simulink library "slctrlblks"  (Simulink 7.6)
settings: Solver=ode45  SolverMode=SingleTasking  StartTime=0.0  StopTime=10.0  RelTol=1e-3
undefined symbols (not defined in the file or in its folder): slctrlblkdlgs
libraries: slctrlextras x12, slctrlblks x6
settings Model: Creator=jglass  LastModifiedBy=astother

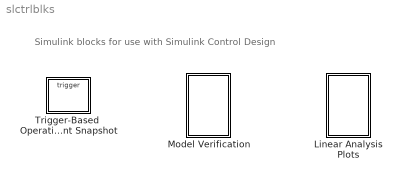
== system slctrlblks ==
  note: Simulink blocks for use with Simulink Control Design
  Linear Analysis Plots : Subsystem
  Model Verification : Subsystem
  Trigger-Based  Operating Point Snapshot : Subsystem  TreatAsAtomicUnit=on  mask(Triggered Operating Condition/Linearization Snapshot){TriggerType=rising}
      mask prompts: TriggerType "Trigger type:"
      mask help: Generate operating points and/or linearizations at triggered events
      mask init:
      | set_param([ gcb '/Trigger'],'TriggerType',TriggerType);
      mask Help: eval('scdguihelp(''trigger_based_operating_point_snapshot_block'',''HelpBrowser'')')
      mask StyleString: popup(rising|falling|either|function-call)

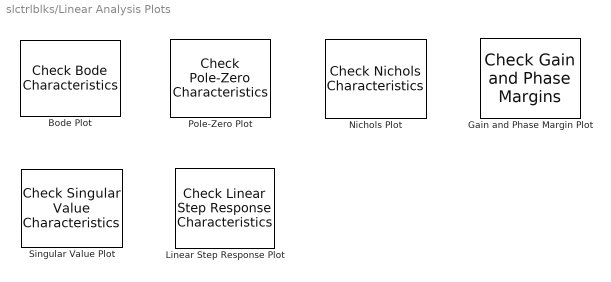
== system slctrlblks/Linear Analysis Plots ==
  Bode Plot : slctrlblks/Model Verification/Check Bode  Characteristics  DialogController=checkpack.createCheckDlg  DialogControllerArgs=DataTag0  SystemSampleTime=-1  LinearizationIOs={}  LinearizeAt=SnapshotTimes  SnapshotTimes=[0]  TriggerType=rising  SampleTime=auto  RateConversionMethod=zoh  PreWarpFreq=10  UseExactDelayModel=off  UseFullBlockNameLabels=off  UseBusSignalLabels=off  enabled=on  stopWhenAssertionFail=off  export=off  ViewDlgPos=[]  OpenViewOnLoad=off  LaunchViewOnOpen=off  EnableUpperBound=off  UpperBoundFrequencies=[]  UpperBoundMagnitudes=[]  EnableLowerBound=off  LowerBoundFrequencies=[]  LowerBoundMagnitudes=[]
  Gain and Phase Margin Plot : slctrlblks/Model Verification/Check Gain and Phase Margins  DialogController=checkpack.createCheckDlg  DialogControllerArgs=DataTag1  SystemSampleTime=-1  LinearizationIOs={}  LinearizeAt=SnapshotTimes  SnapshotTimes=[0]  TriggerType=rising  SampleTime=auto  RateConversionMethod=zoh  PreWarpFreq=10  UseExactDelayModel=off  UseFullBlockNameLabels=off  UseBusSignalLabels=off  enabled=on  stopWhenAssertionFail=off  export=off  ViewDlgPos=[]  LaunchViewOnOpen=off  OpenViewOnLoad=off  EnableMargins=off  GainMargin=[]  PhaseMargin=[]  PlotType=bode  FeedbackSign=-1
      settings: SaveToWorkspace=off  SaveName=sys
  Linear Step Response Plot : slctrlblks/Model Verification/Check Linear Step Response Characteristics  DialogController=checkpack.createCheckDlg  DialogControllerArgs=DataTag2  SystemSampleTime=-1  LinearizationIOs={}  LinearizeAt=SnapshotTimes  SnapshotTimes=[0]  TriggerType=rising  SampleTime=auto  RateConversionMethod=zoh  PreWarpFreq=10  UseExactDelayModel=off  UseFullBlockNameLabels=off  UseBusSignalLabels=off  enabled=on  stopWhenAssertionFail=off  export=off  ViewDlgPos=[]  OpenViewOnLoad=off  LaunchViewOnOpen=off  EnableStepResponseBound=off  FinalValue=[]  RiseTime=[]  PercentRise=[]  SettlingTime=[]  PercentSettling=[]  PercentOvershoot=[]  PercentUndershoot=[]
      settings: SaveToWorkspace=off  SaveName=sys
  Nichols Plot : slctrlblks/Model Verification/Check Nichols Characteristics  DialogController=checkpack.createCheckDlg  DialogControllerArgs=DataTag3  SystemSampleTime=-1  LinearizationIOs={}  LinearizeAt=SnapshotTimes  SnapshotTimes=[0]  TriggerType=rising  SampleTime=auto  RateConversionMethod=zoh  PreWarpFreq=10  UseExactDelayModel=off  UseFullBlockNameLabels=off  UseBusSignalLabels=off  enabled=on  stopWhenAssertionFail=off  export=off  ViewDlgPos=[]  LaunchViewOnOpen=off  OpenViewOnLoad=off  EnableMargins=off  GainMargin=[]  PhaseMargin=[]  EnableGainPhaseBound=off  GainPhaseBoundType={'upper'}  OLPhases=[]  OLGains=[]  EnableCLPeakGain=off  CLPeakGain=[]  FeedbackSign=-1
      settings: SaveToWorkspace=off  SaveName=sys
  Pole-Zero Plot : slctrlblks/Model Verification/Check Pole-Zero Characteristics  DialogController=checkpack.createCheckDlg  DialogControllerArgs=DataTag4  SystemSampleTime=-1  LinearizationIOs={}  LinearizeAt=SnapshotTimes  SnapshotTimes=[0]  TriggerType=rising  SampleTime=auto  RateConversionMethod=zoh  PreWarpFreq=10  UseExactDelayModel=off  UseFullBlockNameLabels=off  UseBusSignalLabels=off  enabled=on  stopWhenAssertionFail=off  export=off  ViewDlgPos=[]  LaunchViewOnOpen=off  OpenViewOnLoad=off  EnableSettlingTime=off  SettlingTime=[]  EnablePercentOvershoot=off  PercentOvershoot=[]  EnableDampingRatio=off  DampingRatio=[]  EnableNaturalFrequency=off  NaturalFrequencyBound=>=  NaturalFrequency=[]
      settings: SaveToWorkspace=off  SaveName=sys
  Singular Value Plot : slctrlblks/Model Verification/Check Singular Value Characteristics  DialogController=checkpack.createCheckDlg  DialogControllerArgs=DataTag5  SystemSampleTime=-1  LinearizationIOs={}  LinearizeAt=SnapshotTimes  SnapshotTimes=[0]  TriggerType=rising  SampleTime=auto  RateConversionMethod=zoh  PreWarpFreq=10  UseExactDelayModel=off  UseFullBlockNameLabels=off  UseBusSignalLabels=off  enabled=on  stopWhenAssertionFail=off  export=off  LaunchViewOnOpen=off  ViewDlgPos=[]  OpenViewOnLoad=off  EnableUpperBound=off  UpperBoundFrequencies=[]  UpperBoundMagnitudes=[]  EnableLowerBound=off  LowerBoundFrequencies=[]  LowerBoundMagnitudes=[]
      settings: SaveToWorkspace=off  SaveName=sys

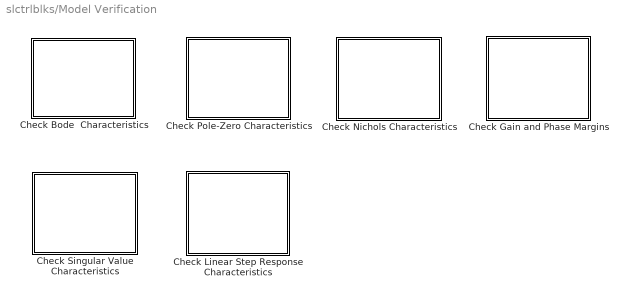
== system slctrlblks/Model Verification ==
  Check Bode  Characteristics : Subsystem  InstantiateOnLoad=on  DialogController=checkpack.createCheckDlg  DialogControllerArgs=DataTag6  LoadFcn=slctrlblkdlgs.absCheckFrequencyDlg.loadBlkFcn(gcb)  mask(Checks_Bode){SaveToWorkspace=off, SaveName=sys, LinearizationIOs={}, LinearizeAt=SnapshotTimes, SnapshotTimes=[0], TriggerType=rising, ZeroCross=on, SampleTime=auto, RateConversionMethod=zoh, PreWarpFreq=10, UseExactDelayModel=off, UseFullBlockNameLabels=off, UseBusSignalLabels=off, enabled=on, callback=, stopWhenAssertionFail=off, export=off, ViewDlgPos=[], OpenViewOnLoad=off, LaunchViewOnOpen=off, FrequencyUnits=, MagnitudeUnits=, PhaseUnits=, EnableUpperBound=on, UpperBoundFrequencies=[10 100], UpperBoundMagnitudes=[-20 -20], EnableLowerBound=on, LowerBoundFrequencies=[0.1 1], LowerBoundMagnitudes=[20 20]}
      mask prompts: SaveToWorkspace "Save data to workspace"; SaveName "Variable name:"; LinearizationIOs "Linearization IOs"; LinearizeAt "Linearize:"; SnapshotTimes "Snapshot times:"; TriggerType "Trigger type:"; ZeroCross "Enable zero-crossing detection"; SampleTime "Sample time:"; RateConversionMethod "Sample time conversion method"; PreWarpFreq "Prewarp frequency"; UseExactDelayModel "Use exact delays"; UseFullBlockNameLabels "Use full block name to label model I/O"; UseBusSignalLabels "Use bus signal nems to label model IO"; enabled "Enable assertion"; callback "Simulation callback when assertion fails (optional):"; stopWhenAssertionFail "Stop simulation when assertion fails"; export "Output assertion signal"; OpenViewOnLoad "Open view when loading"; LaunchViewOnOpen "Launch view on open"; EnableUpperBound "Upper magnitude bound"; UpperBoundFrequencies "Frequencies (Hz):"; UpperBoundMagnitudes "Magnitudes (db):"; EnableLowerBound "Lower magnitude bound"; LowerBoundFrequencies "Frequencies (Hz):"; LowerBoundMagnitudes "Magnitudes (db):"
      mask init:
      | slctrlblkdlgs.CheckBodeDlg.configBlk(gcbh)
      settings: CopyFcn=slctrlblkdlgs.absCheckFrequencyDlg.copyBlkFcn(gcb)  OpenFcn=checkpack.absCheckDlg.openBlkFcn(gcbh)
      mask Help: eval('scdguihelp(''bode_plot_block'',''HelpBrowser'')')
      mask StyleString: checkbox,edit,edit,popup(SnapshotTimes|ExternalTrigger),edit,popup(rising|falling),checkbox,edit,popup(zoh|tustin|prewarp|upsampling_zoh|upsampling_tustin|upsampling_prewarp),edit,checkbox,checkbox,checkbox,checkbox,edit,checkbox,checkbox,edit,checkbox,checkbox,edit,edit,edit,checkbox,edit,edit,checkbox,edit,edit
      mask TabNameString: Logging,Logging,Linearizations,Linearizations,Linearizations,Linearizations,Linearizations,Linearizations,Linearizations,Linearizations,Linearizations,Linearizations,Linearizations,Assertion,Assertion,Assertion,Assertion,Misc.,Misc.,Misc,Misc,Misc,Misc,Bounds,Bounds,Bounds,Bounds,Bounds,Bounds
      mask Display: image(imread('C:\Sandbox\Acontrol_08042010\matlab\toolbox\slcontrol\slctrlutil\resources\CheckBodeIcon.bmp','bmp'),'center');
  Check Gain and Phase Margins : Subsystem  InstantiateOnLoad=on  DialogController=checkpack.createCheckDlg  DialogControllerArgs=DataTag7  LoadFcn=slctrlblkdlgs.absCheckFrequencyDlg.loadBlkFcn(gcb)  mask(Checks_Margins){SaveToWorkspace=off, SaveName=sys, LinearizationIOs={}, LinearizeAt=SnapshotTimes, SnapshotTimes=[0], TriggerType=rising, ZeroCross=on, SampleTime=auto, RateConversionMethod=zoh, PreWarpFreq=10, UseExactDelayModel=off, UseFullBlockNameLabels=off, UseBusSignalLabels=off, enabled=on, callback=, stopWhenAssertionFail=off, export=off, ViewDlgPos=[], LaunchViewOnOpen=off, OpenViewOnLoad=off, FrequencyUnits=, MagnitudeUnits=, PhaseUnits=, EnableMargins=on, GainMargin=20, PhaseMargin=30, PlotType=bode, FeedbackSign=-1}
      mask prompts: SaveToWorkspace "Save data to workspace"; SaveName "Variable name:"; LinearizationIOs "Linearization IOs"; LinearizeAt "Linearize:"; SnapshotTimes "Snapshot times:"; TriggerType "Trigger type:"; ZeroCross "Enable zero-crossing detection"; SampleTime "Sample time:"; RateConversionMethod "Sample time rate conversion method"; PreWarpFreq "Prewarp frequency"; UseExactDelayModel "Use exact delays"; UseFullBlockNameLabels "Use full block name to label model I/O"; UseBusSignalLabels "Use bus signal names to label model I/O"; enabled "Enable assertion"; callback "Simulation callback when assertion fails"; stopWhenAssertionFail "Stop simulation when assertion fails"; export "Output assertion signal"; LaunchViewOnOpen "Launch view on open"; OpenViewOnLoad "Open view when loading"; EnableMargins "Enforce Gain & Phase margins"; GainMargin "Gain margin (db) >"; PhaseMargin "Phase margin (deg) >"; PlotType "Plot type"; FeedbackSign "Feedback sign"
      mask init:
      | slctrlblkdlgs.CheckMarginsDlg.configBlk(gcbh)
      settings: CopyFcn=slctrlblkdlgs.absCheckFrequencyDlg.copyBlkFcn(gcb)  OpenFcn=checkpack.absCheckDlg.openBlkFcn(gcbh)
      mask Help: eval('scdguihelp(''gain_phase_margin_plot_block'',''HelpBrowser'')')
      mask StyleString: checkbox,edit,edit,popup(SnapshotTimes|ExternalTrigger),edit,popup(rising|falling),checkbox,edit,popup(zoh|tustin|prewarp|upsampling_zoh|upsampling_tustin|upsampling_prewarp),edit,checkbox,checkbox,checkbox,checkbox,edit,checkbox,checkbox,edit,checkbox,checkbox,edit,edit,edit,checkbox,edit,edit,popup(bode|nichols|nyquist|table),popup(-1|+1)
      mask TabNameString: Logging,Logging,Linearizations,Linearizations,Linearizations,Linearizations,Linearizations,Linearizations,Linearizations,Linearizations,Linearizations,Linearizations,Linearizations,Assertion,Assertion,Assertion,Assertion,Misc,Misc,Misc,Misc,Misc,Misc,Bounds,Bounds,Bounds,Bounds,Bounds
      mask Display: image(imread('C:\Sandbox\Acontrol_08042010\matlab\toolbox\slcontrol\slctrlutil\resources\CheckMarginsIcon.bmp','bmp'),'center');
  Check Linear Step Response Characteristics : Subsystem  InstantiateOnLoad=on  DialogController=checkpack.createCheckDlg  DialogControllerArgs=DataTag8  LoadFcn=slctrlblkdlgs.absCheckFrequencyDlg.loadBlkFcn(gcb)  mask(Checks_LinearStepResponse){SaveToWorkspace=off, SaveName=sys, LinearizationIOs={}, LinearizeAt=SnapshotTimes, SnapshotTimes=[0], TriggerType=rising, ZeroCross=on, SampleTime=auto, RateConversionMethod=zoh, PreWarpFreq=10, UseExactDelayModel=off, UseFullBlockNameLabels=off, UseBusSignalLabels=off, enabled=on, callback=, stopWhenAssertionFail=off, export=off, ViewDlgPos=[], OpenViewOnLoad=off, LaunchViewOnOpen=off, FrequencyUnits=, MagnitudeUnits=, PhaseUnits=, EnableStepResponseBound=on, FinalValue=1, RiseTime=5, PercentRise=80, SettlingTime=7, PercentSettling=1, PercentOvershoot=10, PercentUndershoot=1}
      mask prompts: SaveToWorkspace "Save data to workspace"; SaveName "Variable name:"; LinearizationIOs "Linearization IOs"; LinearizeAt "Linearize:"; SnapshotTimes "Snapshot times:"; TriggerType "Trigger type:"; ZeroCross "Enable zero-crossing detection"; SampleTime "Sample time:"; RateConversionMethod "Sample time conversion method"; PreWarpFreq "Prewarp frequency"; UseExactDelayModel "Use exact delays"; UseFullBlockNameLabels "Use full block name to label Model I/Os"; UseBusSignalLabels "Use bus signal names to label model I/Os"; enabled "Enable assertion"; callback "Simulation callback when assertion fails"; stopWhenAssertionFail "Stop simulation when assertion fails"; export "Output assertion signal"; OpenViewOnLoad "Open view when loading"; LaunchViewOnOpen "Launch view on open"; EnableStepResponseBound "Enforce Step Response bound"; FinalValue "Final step value:"; RiseTime "Rise time:"; PercentRise "Percentage rise:"; SettlingTime "Settling time:"; PercentSettling "Percentage settling:"; PercentOvershoot "Percentage overshoot:"; PercentUndershoot "Percentage undershoot:"
      mask init:
      | slctrlblkdlgs.CheckLinStepDlg.configBlk(gcbh)
      settings: CopyFcn=slctrlblkdlgs.absCheckFrequencyDlg.copyBlkFcn(gcb)  OpenFcn=checkpack.absCheckDlg.openBlkFcn(gcbh)
      mask Help: eval('scdguihelp(''step_response_plot_block'',''HelpBrowser'')')
      mask StyleString: checkbox,edit,edit,popup(SnapshotTimes|ExternalTrigger),edit,popup(rising|falling),checkbox,edit,popup(zoh|tustin|prewarp|upsampling_zoh|upsampling_tustin|upsampling_prewarp),edit,checkbox,checkbox,checkbox,checkbox,edit,checkbox,checkbox,edit,checkbox,checkbox,edit,edit,edit,checkbox,edit,edit,edit,edit,edit,edit,edit
      mask TabNameString: Logging,Logging,Linearizations,Linearizations,Linearizations,Linearizations,Linearizations,Linearizations,Linearizations,Linearizations,Linearizations,Linearizations,Linearizations,Assertion,Assertion,Assertion,Assertion,Misc,Misc,Misc,Misc,Misc,Misc,Bounds,Bounds,Bounds,Bounds,Bounds,Bounds,Bounds,Bounds
      mask Display: image(imread('C:\Sandbox\Acontrol_08042010\matlab\toolbox\slcontrol\slctrlutil\resources\CheckLinStepIcon.bmp','bmp'),'center');
  Check Nichols Characteristics : Subsystem  InstantiateOnLoad=on  DialogController=checkpack.createCheckDlg  DialogControllerArgs=DataTag9  LoadFcn=slctrlblkdlgs.absCheckFrequencyDlg.loadBlkFcn(gcb)  mask(Checks_Nichols){SaveToWorkspace=off, SaveName=sys, LinearizationIOs={}, LinearizeAt=SnapshotTimes, SnapshotTimes=[0], TriggerType=rising, ZeroCross=on, SampleTime=auto, RateConversionMethod=zoh, PreWarpFreq=10, UseExactDelayModel=off, UseFullBlockNameLabels=off, UseBusSignalLabels=off, enabled=on, callback=, stopWhenAssertionFail=off, export=off, ViewDlgPos=[], LaunchViewOnOpen=off, OpenViewOnLoad=off, FrequencyUnits=, MagnitudeUnits=, PhaseUnits=, EnableMargins=on, GainMargin=20, PhaseMargin=30, EnableGainPhaseBound=off, GainPhaseBoundType={'upper'}, OLPhases=[], OLGains=[], EnableCLPeakGain=off, CLPeakGain=[], FeedbackSign=-1}
      mask prompts: SaveToWorkspace "Save data to workspace"; SaveName "Variable name:"; LinearizationIOs "Linearization IOs"; LinearizeAt "Linearize:"; SnapshotTimes "Snapshot times:"; TriggerType "Trigger type:"; ZeroCross "Enable zero-crossing detection"; SampleTime "Sample time:"; RateConversionMethod "Sample time conversion method"; PreWarpFreq "Prewarp frequency"; UseExactDelayModel "Use exact delays"; UseFullBlockNameLabels "Use full block name to label model I/O"; UseBusSignalLabels "Use bus signal names to label model I/O"; enabled "Enable assertion"; callback "Simulation callback when assertion fails"; stopWhenAssertionFail "Stop simulation when assertion fails"; export "Output assertion signal"; LaunchViewOnOpen "Launch view on open"; OpenViewOnLoad "Open view when loading"; EnableMargins "Enforce Gain & Phase margins"; GainMargin "Gain margin (db) >"; PhaseMargin "Phase margin (deg) >"; EnableGainPhaseBound "Gain-Phase bound"; GainPhaseBoundType "Type:"; OLPhases "Open-loop phases (deg)"; OLGains "Open-loop gains (db)"; EnableCLPeakGain "Closed-loop peak gain bound"; CLPeakGain "Closed-loop peak gain (db) <"; FeedbackSign "Feedback sign"
      mask init:
      | slctrlblkdlgs.CheckNicholsDlg.configBlk(gcbh)
      settings: CopyFcn=slctrlblkdlgs.absCheckFrequencyDlg.copyBlkFcn(gcb)  OpenFcn=checkpack.absCheckDlg.openBlkFcn(gcbh)
      mask Help: eval('scdguihelp(''nichols_plot_block'',''HelpBrowser'')')
      mask StyleString: checkbox,edit,edit,popup(SnapshotTimes|ExternalTrigger),edit,popup(rising|falling),checkbox,edit,popup(zoh|tustin|prewarp|upsampling_zoh|upsampling_tustin|upsampling_prewarp),edit,checkbox,checkbox,checkbox,checkbox,edit,checkbox,checkbox,edit,checkbox,checkbox,edit,edit,edit,checkbox,edit,edit,checkbox,edit,edit,edit,checkbox,edit,popup(-1|+1)
      mask TabNameString: Logging,Logging,Linearizations,Linearizations,Linearizations,Linearizations,Linearizations,Linearizations,Linearizations,Linearizations,Linearizations,Linearizations,Linearizations,Assertion,Assertion,Assertion,Assertion,Misc,Misc,Misc,Misc,Misc,Misc,Bounds,Bounds,Bounds,Bounds,Bounds,Bounds,Bounds,Bounds,Bounds,Bounds
      mask Display: image(imread('C:\Sandbox\Acontrol_08042010\matlab\toolbox\slcontrol\slctrlutil\resources\CheckNicholsIcon.bmp','bmp'),'center');
  Check Pole-Zero Characteristics : Subsystem  InstantiateOnLoad=on  DialogController=checkpack.createCheckDlg  DialogControllerArgs=DataTag10  LoadFcn=slctrlblkdlgs.absCheckFrequencyDlg.loadBlkFcn(gcb)  mask(Checks_PZMap){SaveToWorkspace=off, SaveName=sys, LinearizationIOs={}, LinearizeAt=SnapshotTimes, SnapshotTimes=[0], TriggerType=rising, ZeroCross=on, SampleTime=auto, RateConversionMethod=zoh, PreWarpFreq=10, UseExactDelayModel=off, UseFullBlockNameLabels=off, UseBusSignalLabels=off, enabled=on, callback=, stopWhenAssertionFail=off, export=off, ViewDlgPos=[], LaunchViewOnOpen=off, OpenViewOnLoad=off, FrequencyUnits=, MagnitudeUnits=, PhaseUnits=, EnableSettlingTime=on, SettlingTime=1, EnablePercentOvershoot=on, PercentOvershoot=10, EnableDampingRatio=off, DampingRatio=[], EnableNaturalFrequency=off, NaturalFrequencyBound=>=, NaturalFrequency=[]}
      mask prompts: SaveToWorkspace "Save data to workspace"; SaveName "Variable name:"; LinearizationIOs "Linearization IOs"; LinearizeAt "Linearize:"; SnapshotTimes "Snapshot times:"; TriggerType "Trigger type:"; ZeroCross "Enable zero-crossing detection"; SampleTime "Sample time:"; RateConversionMethod "Sample time conversion method"; PreWarpFreq "Prewarp frequency"; UseExactDelayModel "Use exact delays"; UseFullBlockNameLabels "Use full block name to label model I/O"; UseBusSignalLabels "Use bus signal names to label model I/O"; enabled "Enable assertion"; callback "Simulation callback when assertion fails"; stopWhenAssertionFail "Stop simulation when assertion fails"; export "Output assertion signal"; LaunchViewOnOpen "Launch view on open"; OpenViewOnLoad "Open view when loading"; EnableSettlingTime "Settling time bound"; SettlingTime "Settling time (sec) <"; EnablePercentOvershoot "Overshoot bound"; PercentOvershoot "Percent overshoot <"; EnableDampingRatio "Damping ratio bound"; DampingRatio "Damping ratio <"; EnableNaturalFrequency "Natural frequency bound"; NaturalFrequencyBound "Natural frequency bound type"; NaturalFrequency "Natural frequency"
      mask init:
      | slctrlblkdlgs.CheckPZMapDlg.configBlk(gcbh)
      settings: CopyFcn=slctrlblkdlgs.absCheckFrequencyDlg.copyBlkFcn(gcb)  OpenFcn=checkpack.absCheckDlg.openBlkFcn(gcbh)
      mask Help: eval('scdguihelp(''pole_zero_plot_block'',''HelpBrowser'')')
      mask StyleString: checkbox,edit,edit,popup(SnapshotTimes|ExternalTrigger),edit,popup(rising|falling),checkbox,edit,popup(zoh|tustin|prewarp|upsampling_zoh|upsampling_tustin|upsampling_prewarp),edit,checkbox,checkbox,checkbox,checkbox,edit,checkbox,checkbox,edit,checkbox,checkbox,edit,edit,edit,checkbox,edit,checkbox,edit,checkbox,edit,checkbox,popup(>=|<=),edit
      mask TabNameString: Logging,Logging,Linearizations,Linearizations,Linearizations,Linearizations,Linearizations,Linearizations,Linearizations,Linearizations,Linearizations,Linearizations,Linearizations,Assertion,Assertion,Assertion,Assertion,Misc.,Misc.,Misc.,Misc.,Misc.,Misc.,Bounds,Bounds,Bounds,Bounds,Bounds,Bounds,Bounds,Bounds,Bounds
      mask Display: image(imread('C:\Sandbox\Acontrol_08042010\matlab\toolbox\slcontrol\slctrlutil\resources\CheckPZMapIcon.bmp','bmp'),'center');
  Check Singular Value Characteristics : Subsystem  InstantiateOnLoad=on  DialogController=checkpack.createCheckDlg  DialogControllerArgs=DataTag11  LoadFcn=slctrlblkdlgs.absCheckFrequencyDlg.loadBlkFcn(gcb)  mask(Checks_Sigma){SaveToWorkspace=off, SaveName=sys, LinearizationIOs={}, LinearizeAt=SnapshotTimes, SnapshotTimes=[0], TriggerType=rising, ZeroCross=on, SampleTime=auto, RateConversionMethod=zoh, PreWarpFreq=10, UseExactDelayModel=off, UseFullBlockNameLabels=off, UseBusSignalLabels=off, enabled=on, callback=, stopWhenAssertionFail=off, export=off, LaunchViewOnOpen=off, ViewDlgPos=[], OpenViewOnLoad=off, FrequencyUnits=, MagnitudeUnits=, PhaseUnits=, EnableUpperBound=on, UpperBoundFrequencies=[0.1 100], UpperBoundMagnitudes=[0 0], EnableLowerBound=off, LowerBoundFrequencies=[], LowerBoundMagnitudes=[]}
      mask prompts: SaveToWorkspace "Save data to workspace"; SaveName "Variable name:"; LinearizationIOs "Linearization IOs"; LinearizeAt "Linearize:"; SnapshotTimes "Snapshot times:"; TriggerType "Trigger type:"; ZeroCross "Enable zero-crossing detection"; SampleTime "Sample time:"; RateConversionMethod "Sample time conversion method"; PreWarpFreq "Prewarp frequency"; UseExactDelayModel "Use exact delays"; UseFullBlockNameLabels "Use full block name to label model I/Os"; UseBusSignalLabels "Use bus signal names to label model I/Os"; enabled "Enable assertion"; callback "Simulation callback when assertion fails (optional)"; stopWhenAssertionFail "Stop simulation when assertion fails"; export "Output assertion signal"; LaunchViewOnOpen "Launch view on open"; OpenViewOnLoad "Open view when loading"; EnableUpperBound "Upper magnitude bound"; UpperBoundFrequencies "Frequencies (Hz):"; UpperBoundMagnitudes "Magnitudes (dB):"; EnableLowerBound "Lower magnitude bound"; LowerBoundFrequencies "Frequencies (Hz):"; LowerBoundMagnitudes "Magnitudes (dB):"
      mask init:
      | slctrlblkdlgs.CheckSVDDlg.configBlk(gcbh)
      settings: CopyFcn=slctrlblkdlgs.absCheckFrequencyDlg.copyBlkFcn(gcb)  OpenFcn=checkpack.absCheckDlg.openBlkFcn(gcbh)
      mask Help: eval('scdguihelp(''max_singular_value_plot_block'',''HelpBrowser'')')
      mask StyleString: checkbox,edit,edit,popup(SnapshotTimes|ExternalTrigger),edit,popup(rising|falling),checkbox,edit,popup(zoh|tustin|prewarp|upsampling_zoh|upsampling_tustin|upsampling_prewarp),edit,checkbox,checkbox,checkbox,checkbox,edit,checkbox,checkbox,checkbox,edit,checkbox,edit,edit,edit,checkbox,edit,edit,checkbox,edit,edit
      mask TabNameString: Logging,Logging,Linearizations,Linearizations,Linearizations,Linearizations,Linearizations,Linearizations,Linearizations,Linearizations,Linearizations,Linearizations,Linearizations,Assertion,Assertion,Assertion,Assertion,Misc,Misc,Misc,Misc,Misc,Misc,Bounds,Bounds,Bounds,Bounds,Bounds,Bounds
      mask Display: image(imread('C:\Sandbox\Acontrol_08042010\matlab\toolbox\slcontrol\slctrlutil\resources\CheckSVDIcon.bmp','bmp'),'center');

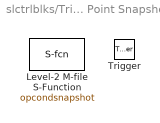
== system slctrlblks/Trigger-Based  Operating Point Snapshot ==
  Trigger : TriggerPort
  Level-2 M-file S-Function : M-S-Function  FunctionName=opcondsnapshot

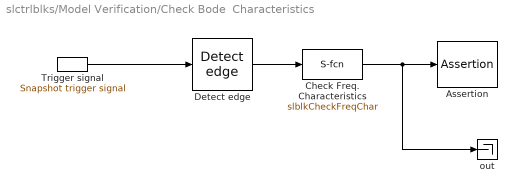
== system slctrlblks/Model Verification/Check Bode  Characteristics ==
  Assertion : Assertion  Enabled=on  AssertionFailFcn=eval(callback)  StopWhenAssertionFail=off
  Check Freq. Characteristics : M-S-Function  FunctionName=slblkCheckFreqChar
  Detect edge : slctrlextras/Detect edge  SystemSampleTime=-1  TriggerType=rising
  Trigger signal : slctrlextras/Snapshot trigger signal  SystemSampleTime=-1
  out : Terminator
  wires:
  Trigger signal/1 -> Detect edge/1
  Detect edge/1 -> Check Freq. Characteristics/1
  Check Freq. Characteristics/1 -> out/1, Assertion/1

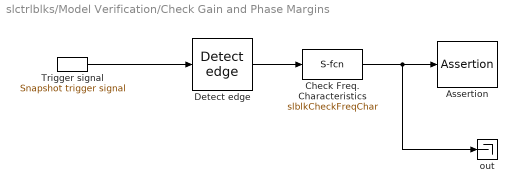
== system slctrlblks/Model Verification/Check Gain and Phase Margins ==
  Assertion : Assertion  Enabled=on  AssertionFailFcn=eval(callback)  StopWhenAssertionFail=off
  Check Freq. Characteristics : M-S-Function  FunctionName=slblkCheckFreqChar
  Detect edge : slctrlextras/Detect edge  SystemSampleTime=-1  TriggerType=rising
  Trigger signal : slctrlextras/Snapshot trigger signal  SystemSampleTime=-1
  out : Terminator
  wires:
  Trigger signal/1 -> Detect edge/1
  Detect edge/1 -> Check Freq. Characteristics/1
  Check Freq. Characteristics/1 -> out/1, Assertion/1

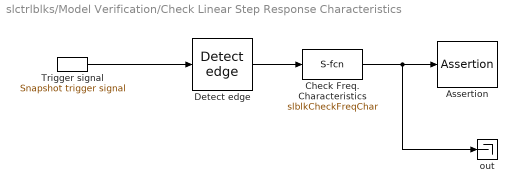
== system slctrlblks/Model Verification/Check Linear Step Response Characteristics ==
  Assertion : Assertion  Enabled=on  AssertionFailFcn=eval(callback)  StopWhenAssertionFail=off
  Check Freq. Characteristics : M-S-Function  FunctionName=slblkCheckFreqChar
  Detect edge : slctrlextras/Detect edge  SystemSampleTime=-1  TriggerType=rising
  Trigger signal : slctrlextras/Snapshot trigger signal  SystemSampleTime=-1
  out : Terminator
  wires:
  Trigger signal/1 -> Detect edge/1
  Detect edge/1 -> Check Freq. Characteristics/1
  Check Freq. Characteristics/1 -> out/1, Assertion/1

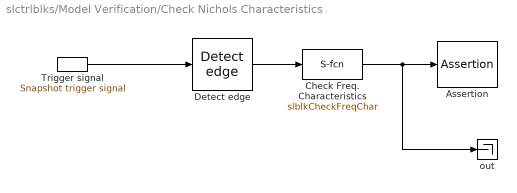
== system slctrlblks/Model Verification/Check Nichols Characteristics ==
  Assertion : Assertion  Enabled=on  AssertionFailFcn=eval(callback)  StopWhenAssertionFail=off
  Check Freq. Characteristics : M-S-Function  FunctionName=slblkCheckFreqChar
  Detect edge : slctrlextras/Detect edge  SystemSampleTime=-1  TriggerType=rising
  Trigger signal : slctrlextras/Snapshot trigger signal  SystemSampleTime=-1
  out : Terminator
  wires:
  Trigger signal/1 -> Detect edge/1
  Detect edge/1 -> Check Freq. Characteristics/1
  Check Freq. Characteristics/1 -> Assertion/1, out/1

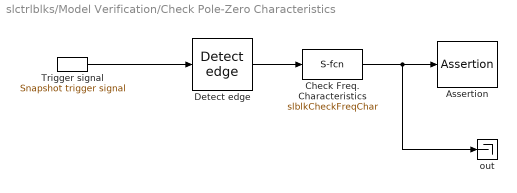
== system slctrlblks/Model Verification/Check Pole-Zero Characteristics ==
  Assertion : Assertion  Enabled=on  AssertionFailFcn=eval(callback)  StopWhenAssertionFail=off
  Check Freq. Characteristics : M-S-Function  FunctionName=slblkCheckFreqChar
  Detect edge : slctrlextras/Detect edge  SystemSampleTime=-1  TriggerType=rising
  Trigger signal : slctrlextras/Snapshot trigger signal  SystemSampleTime=-1
  out : Terminator
  wires:
  Trigger signal/1 -> Detect edge/1
  Detect edge/1 -> Check Freq. Characteristics/1
  Check Freq. Characteristics/1 -> Assertion/1, out/1

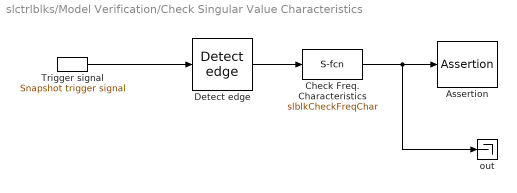
== system slctrlblks/Model Verification/Check Singular Value Characteristics ==
  Assertion : Assertion  Enabled=on  AssertionFailFcn=eval(callback)  StopWhenAssertionFail=off
  Check Freq. Characteristics : M-S-Function  FunctionName=slblkCheckFreqChar
  Detect edge : slctrlextras/Detect edge  SystemSampleTime=-1  TriggerType=rising
  Trigger signal : slctrlextras/Snapshot trigger signal  SystemSampleTime=-1
  out : Terminator
  wires:
  Trigger signal/1 -> Detect edge/1
  Detect edge/1 -> Check Freq. Characteristics/1
  Check Freq. Characteristics/1 -> Assertion/1, out/1
